simulink model "array"  (R2014a)
settings: Solver=ode45  StartTime=0.0  StopTime=2*Tgrid  RelTol=1e-3
values from neighbouring files (symbols this model uses):
  Tgrid = (1 / Fgrid)    (= 0.0166666666667)    [array_init.m]
  Tswitch = [Tswitch; zeros(1,5)]    [array_init.m]
  Vgrid = (sqrt(2)*Vgridrms)    [array_init.m]
undefined symbols (not defined in the file or in its folder): N
libraries: module_switch x12, dspxfrm3 x1, powerlib_meascontrol x1
settings Model: Creator=Taylor  LastModifiedBy=Taylor
settings DataIOCC: LimitDataPoints=off  SaveFinalState=on  SignalLoggingSaveFormat=ModelDataLogs  SaveState=on
settings OptimizationCC: InlineParams=on
settings DebuggingCC: UnderspecifiedInitializationDetection=Classic  MultiTaskDSMMsg=warning  MultiTaskCondExecSysMsg=none
settings RTWCC: IncludeERTFirstTime=on

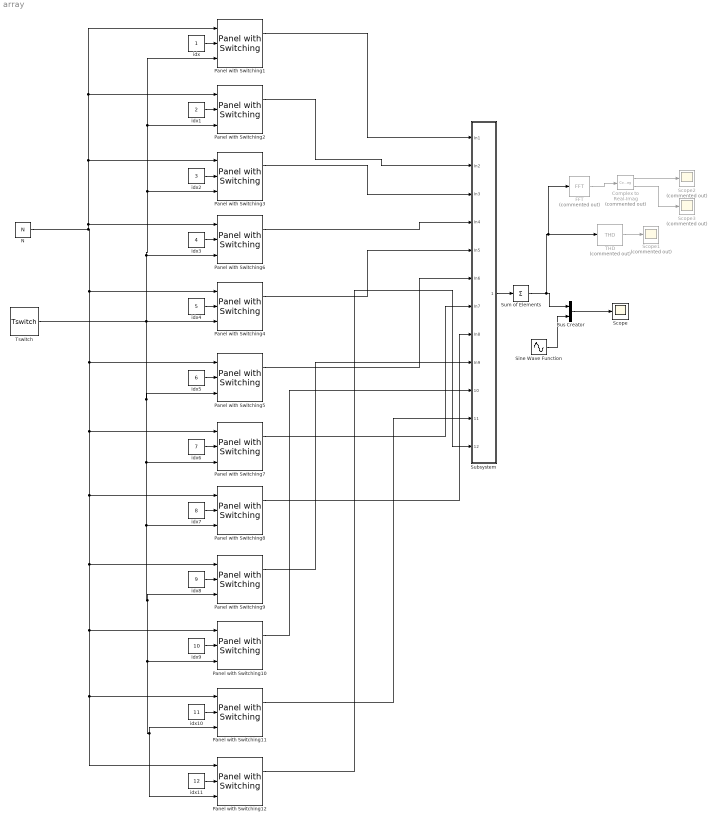
== system array ==
  Bus Creator : BusCreator  Inputs=2
  Complex to Real-Imag : ComplexToRealImag  Commented=on
  FFT : dspxfrm3/FFT  Commented=on  CompMethod=Table lookup  TableOpt=NEW  TableOptActive=Speed  BitRevOrder=off  InheritFFTLength=on  FFTLength=64  WrapInput=on  RowConvenienceOn=on  FFTImplementation=Auto  SkipNorm=off  firstCoeffDataTypeStr=Inherit: Same word length as input  firstCoeffLastDataTypeStr=Inherit: Same word length as input  outputMin=[]  outputMax=[]  roundingMode=Floor  overflowMode=off
  N : Constant  Value=N
  Panel with Switching{1..12} (12 alike) : module_switch/Panel with Switching
  Scope : Scope
      settings: TimeRange=0.0166667  YMin=-40  YMax=180
  Scope1 : Scope  Commented=on
      settings: TimeRange=0.0166667  YMin=0.04275  YMax=0.04335  SaveName=ScopeData2
  Scope2 : Scope  Commented=on
      settings: TimeRange=0.0166667  YMin=-142.5  YMax=-112.5  SaveName=ScopeData3
  Scope3 : Scope  Commented=on
      settings: TimeRange=0.0166667  YMin=20  YMax=180  SaveName=ScopeData4
  Sine Wave Function : Sin  Amplitude=Vgrid  Frequency=2*pi/Tgrid  SampleTime=0
  Subsystem : Subsystem
  Sum of Elements : Sum  Inputs=+
  THD : powerlib_meascontrol/Measurements/THD  Commented=on  Freq=Fgrid  Ts=0
  Tswitch : Constant  Value=Tswitch
  idx : Constant
  idx1 : Constant  Value=2
  idx10 : Constant  Value=11
  idx11 : Constant  Value=12
  idx2 : Constant  Value=3
  idx3 : Constant  Value=4
  idx4 : Constant  Value=5
  idx5 : Constant  Value=6
  idx6 : Constant  Value=7
  idx7 : Constant  Value=8
  idx8 : Constant  Value=9
  idx9 : Constant  Value=10
  wires:
  N/1 -> Panel with Switching5/1, Panel with Switching8/1, Panel with Switching9/1, Panel with Switching11/1, Panel with Switching12/1, Panel with Switching10/1, Panel with Switching7/1, Panel with Switching4/1, Panel with Switching3/1, Panel with Switching2/1, Panel with Switching1/1, Panel with Switching6/1
  idx/1 -> Panel with Switching1/2
  Tswitch/1 -> Panel with Switching4/3, Panel with Switching2/3, Panel with Switching1/3, Panel with Switching3/3, Panel with Switching6/3, Panel with Switching12/3, Panel with Switching11/3, Panel with Switching10/3, Panel with Switching9/3, Panel with Switching8/3, Panel with Switching7/3, Panel with Switching5/3
  Sum of Elements/1 -> FFT/1, THD/1, Bus Creator/1
  idx1/1 -> Panel with Switching2/2
  idx3/1 -> Panel with Switching6/2
  idx2/1 -> Panel with Switching3/2
  idx4/1 -> Panel with Switching4/2
  idx5/1 -> Panel with Switching5/2
  idx6/1 -> Panel with Switching7/2
  idx7/1 -> Panel with Switching8/2
  idx8/1 -> Panel with Switching9/2
  idx9/1 -> Panel with Switching10/2
  idx10/1 -> Panel with Switching11/2
  idx11/1 -> Panel with Switching12/2
  Panel with Switching1/1 -> Subsystem/1(In1)
  Panel with Switching2/1 -> Subsystem/2(In2)
  Panel with Switching3/1 -> Subsystem/3(In3)
  Panel with Switching6/1 -> Subsystem/4(In4)
  Panel with Switching4/1 -> Subsystem/5(In5)
  Panel with Switching5/1 -> Subsystem/6(In6)
  Panel with Switching7/1 -> Subsystem/7(In7)
  Panel with Switching8/1 -> Subsystem/8(In8)
  Panel with Switching9/1 -> Subsystem/9(In9)
  Panel with Switching10/1 -> Subsystem/10(In10)
  Panel with Switching11/1 -> Subsystem/11(In11)
  Panel with Switching12/1 -> Subsystem/12(In12)
  Subsystem/1(Out1) -> Sum of Elements/1
  Sine Wave Function/1 -> Bus Creator/2
  Bus Creator/1 -> Scope/1
  THD/1 -> Scope1/1
  FFT/1 -> Complex to Real-Imag/1
  Complex to Real-Imag/1 -> Scope2/1
  Complex to Real-Imag/2 -> Scope3/1

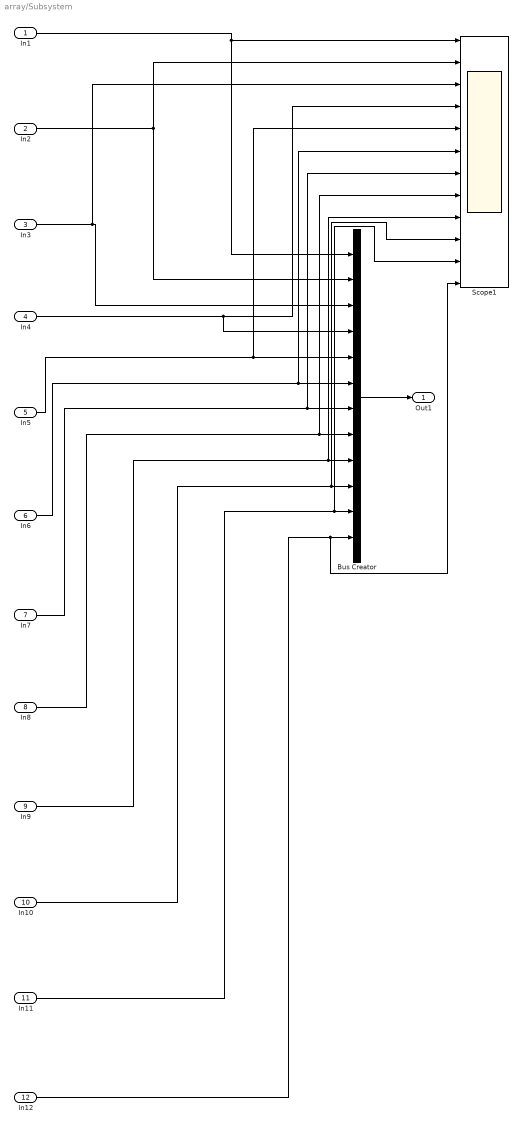
== system array/Subsystem ==
  In1 : Inport
  In2 : Inport  Port=2
  In3 : Inport  Port=3
  In4 : Inport  Port=4
  In5 : Inport  Port=5
  In6 : Inport  Port=6
  In7 : Inport  Port=7
  In8 : Inport  Port=8
  In9 : Inport  Port=9
  In10 : Inport  Port=10
  In11 : Inport  Port=11
  In12 : Inport  Port=12
  Bus Creator : BusCreator  Inputs=12
  Scope1 : Scope  NumInputPorts=12
      settings: TimeRange=0.0333333  YMin=-3~-3~-3~-3~-3~-3~0~0~0~0~0~0  YMax=3~3~3~3~3~3~2.5~2.5~2.5~2.5~2.5~2.5
  Out1 : Outport
  wires:
  Bus Creator/1 -> Out1/1
  In1/1 -> Scope1/1, Bus Creator/1
  In2/1 -> Scope1/2, Bus Creator/2
  In4/1 -> Scope1/4, Bus Creator/4
  In6/1 -> Scope1/6, Bus Creator/6
  In7/1 -> Scope1/7, Bus Creator/7
  In5/1 -> Scope1/5, Bus Creator/5
  In12/1 -> Scope1/12, Bus Creator/12
  In3/1 -> Scope1/3, Bus Creator/3
  In8/1 -> Scope1/8, Bus Creator/8
  In10/1 -> Scope1/10, Bus Creator/10
  In9/1 -> Scope1/9, Bus Creator/9
  In11/1 -> Scope1/11, Bus Creator/11
